simulink model "exp1force_3012"  (R2018b)
settings: Solver=VariableStepAuto  StartTime=0  StopTime=10.0  RelTol=1e-3
values from neighbouring files (symbols this model uses):
  B = 2.5    [exp001_3012.m]
  K = 16    [exp001_3012.m]
  M = 20    [exp001_3012.m]
settings Model: Creator=student  LastModifiedBy=student

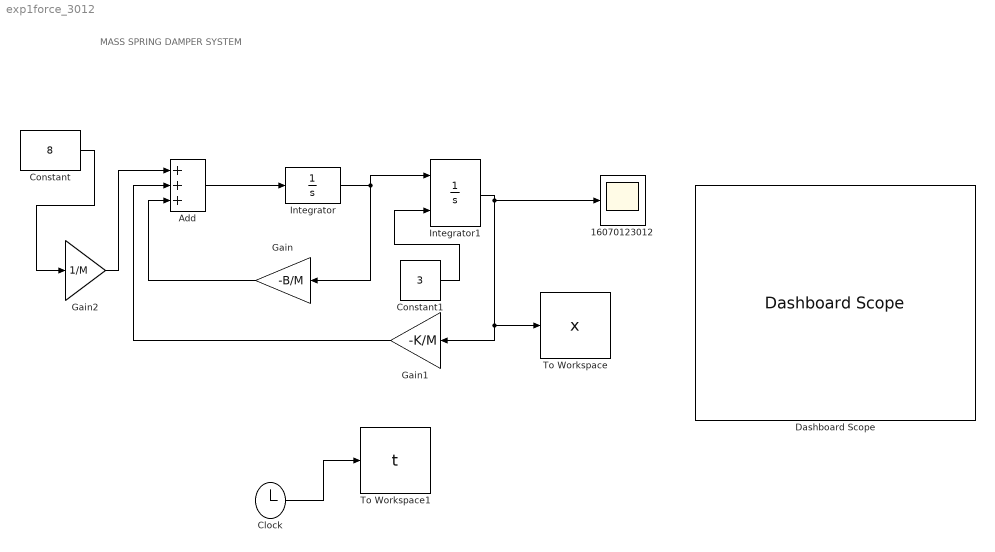
== system exp1force_3012 ==
  note: MASS SPRING DAMPER SYSTEM
  16070123012 : Scope
  Add : Sum  Inputs=+++
  Clock : Clock
  Constant : Constant  Value=8
  Constant1 : Constant  Value=3
  Dashboard Scope : DashboardScope  WebBlockId=22
  Gain : Gain  Gain=-B/M
  Gain1 : Gain  Gain=-K/M
  Gain2 : Gain  Gain=1/M
  Integrator : Integrator
  Integrator1 : Integrator  InitialConditionSource=external  InitialCondition=5
  To Workspace : ToWorkspace  VariableName=x  SampleTime=-1
  To Workspace1 : ToWorkspace  VariableName=t  SaveFormat=Timeseries  SampleTime=-1
  wires:
  Gain2/1 -> Add/1
  Integrator/1 -> Gain/1, Integrator1/1
  Integrator1/1 -> To Workspace/1, Gain1/1, 16070123012/1
  Gain1/1 -> Add/2
  Gain/1 -> Add/3
  Add/1 -> Integrator/1
  Constant/1 -> Gain2/1
  Constant1/1 -> Integrator1/2
  Clock/1 -> To Workspace1/1
